simulink model "BandBlinear"  (Simulink 7.0)
settings: Solver=ode45  StartTime=tstart  StopTime=tstop  RelTol=1e-3
values from neighbouring files (symbols this model uses):
  A = [0 1 0 0; 0 0 -Bb*G 0; 0 0 0 1; -M*G/(J + Jb) 0 0 0]    [BandBinit.m]    (also in EE6283_Final_QuyenHua.m = [-0.5164 1 -0.0717; 1.4168 -0.4932 -1.6450; 0 0 -10]; EE6283_LearningModule1_Problem2_QuyenHua.m = [0 1/L; 1/C -1/(R*C)]; EE6283_M10_CME7p4_QuyenHua.m = [0 1 0 0; 0 0 1 0; 0 0 0 1; -962 -126 -67 -4]; EE6283_M11_CME8p4A_QuyenHua.m = [0 1 0 0; 0 0 1 0; 0 0 0 1; -962 -126 -67 -4])
  B = M / (Jb/R^2 + M)    [BandBfun.m]    (also in BandBinit.m = [0; 0; 0; 1/(J + Jb)]; EE6283_Final_QuyenHua.m = [0; 0; 10]; EE6283_LearningModule1_Problem2_QuyenHua.m = [-1/L; 0]; EE6283_M10_CME7p4_QuyenHua.m = [0; 0; 0; 1])
  x0 = p0 * diag([1 1 -1/Bb/G -1/Bb/G]) * [1; 0; -sqrt(-a0); 0]    [BandBinit.m]    (also in EE6283_M9_CE6p2_QuyenHua.m = [10; 10; 10; 10]; EE6283_M9_CME6p4_QuyenHua.m = [10; 10; 10; 10]; EE6283_M9_NE6p3_QuyenHua.m = [10; 10]; InvPendInit.m = [0 0 0 0])
settings Model: Creator=Doug  LastModifiedBy=Doug
settings DataIOCC: LimitDataPoints=off  SaveOutput=off  SignalLogging=off  SaveTime=off
settings DebuggingCC: SolverPrmCheckMsg=none

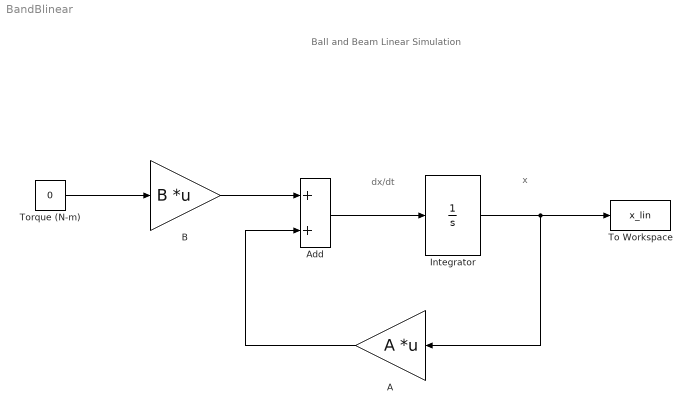
== system BandBlinear ==
  note: Ball and Beam Linear Simulation
  note: dx/dt
  note: x
  A : Gain  Orientation=left  Gain=A  Multiplication=Matrix(K*u)  ParameterDataType=sfix(16)  ParameterScaling=2^0  OutDataType=sfix(16)  OutScaling=2^0
  Add : Sum  OutDataType=sfix(16)  OutScaling=2^-10
  B : Gain  Gain=B  Multiplication=Matrix(K*u)  ParameterDataType=sfix(16)  ParameterScaling=2^0  OutDataType=sfix(16)  OutScaling=2^0
  Integrator : Integrator  InitialCondition=x0
  To Workspace : ToWorkspace  VariableName=x_lin  SampleTime=-1  SaveFormat=Structure With Time
  Torque (N-m) : Constant  Value=0  OutDataType=sfix(16)  OutScaling=2^0
  wires:
  Add/1 -> Integrator/1
  B/1 -> Add/1
  Integrator/1 -> A/1, To Workspace/1
  A/1 -> Add/2
  Torque (N-m)/1 -> B/1
